simulink model "furuta"  (R2025b)
settings: Solver=VariableStepAuto  StartTime=0.0  StopTime=5  FixedStep=0.01  MaxStep=0.01  RelTol=1e-3
values from neighbouring files (symbols this model uses):
  A_i = double( subs( A_i, subs_array(:,1), subs_array(:,2) ) )    [define_dynamics.m]    (also in dynamics.mat = [0 0 0 0 0 0 0 0 74.6600956651 148.711425653 0 0 ... (25 ele)
  A_s = double( subs( A_s, subs_array(:,1), subs_array(:,2) ) )    [define_dynamics.m]    (also in dynamics.mat = [0 0 0 0 0 0 0 0 74.6600956651 -148.711425653 0 0 ... (25 el)
  Abig_i = [ A_i-B_i*K_i          , B_i*K_i ... (first row only)    [create_inverted_ctrl.m]
  B_i = double( subs( B_i, subs_array(:,1), subs_array(:,2) ) )    [define_dynamics.m]    (also in dynamics.mat = [0 0 625 0 0])
  B_s = double( subs( B_s, subs_array(:,1), subs_array(:,2) ) )    [define_dynamics.m]    (also in dynamics.mat = [0 0 625 0 0])
  C = eye( 5, 5 )    [define_dynamics.m]    (also in dynamics.mat = [1 0 0 0 0 0 1 0 0 0 0 0 ... (25 elements, 5x5)])
  C_i = [ 1 0 0 0 0 ... (first row only)    [create_inverted_ctrl.m]    (also in create_inverted_ctrl_dt.m)
  C_s = [ 0 ]    [analyze_linear_dynamics.m]    (also in create_suspended_ctrl.m = [1 0 0 0 0; create_suspended_ctrl_dt.m = [ 1 0 0 0 0; simulink_companion.m = [ 1 0 0 0 0)
  D = zeros( 5, 1 )    [define_dynamics.m]    (also in dynamics.mat = [0 0 0 0 0])
  D_s = zeros(3,1)    [create_suspended_ctrl.m]    (also in create_suspended_ctrl_dt.m = [ 0; simulink_companion.m = zeros( 3, 5 ))
  K_i = place( A_i, B_i, p )    [create_inverted_ctrl.m]    (also in create_inverted_ctrl_dt.m = place( A_i, B_i, pc ))
  K_s = place( A_s, B_s, p )    [analyze_linear_dynamics.m]    (also in create_suspended_ctrl.m = place( A_s, B_s, pc ); simulink_companion.m)
  K_s_nl = K_s    [simulink_companion.m]
  L_i = place( A_i', C_i', p )'    [create_inverted_ctrl.m]    (also in create_inverted_ctrl_dt.m = place( A_i', C_i', po )')
  L_s = place( A_s', C_s', po )'    [create_suspended_ctrl.m]    (also in simulink_companion.m = place( A_s', C_s', p )')
libraries: simulink x1
settings Model: Creator=shara  LastModifiedBy=shara

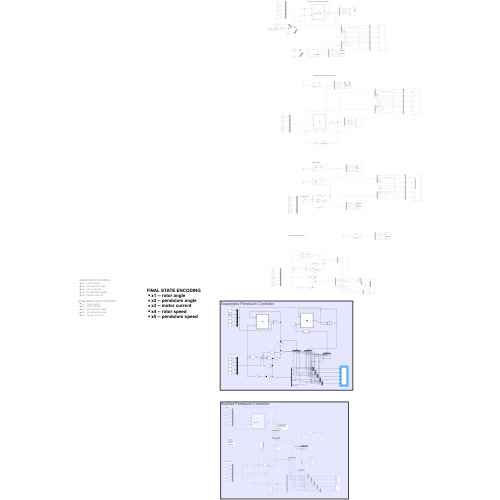
[thumbnail: Simulink's stored preview of the top-level diagram]
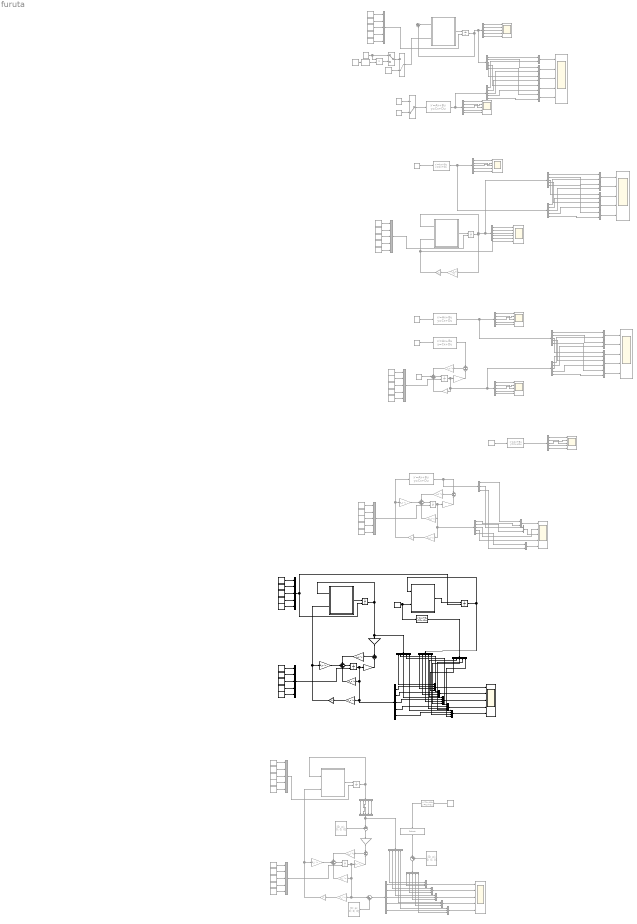
== system furuta ==
  note: $\tilde{x} = x - x_\text{eq}$
  note: LINEAR STATE ENCODING
      | x1 -- rotor angle
      | x2 -- pendulum angle
      | x3 -- rotor speed
      | x4 -- pendulum speed
      | x5 -- motor current
      |
      | NONLINEAR STATE ENCODING
      | x1 -- rotor angle
      | x2 -- rotor speed
      | x3 -- pendulum angle
      | x4 -- pendulum speed
      | x5 -- motor current
  note: NOTE: V_eq = 0, so we don't have to adjust the pertubation
  note: Suspended Pendulum Controller
  note: Observer ICs
  note: State ICs
  note: Combined controller and observer
  note: Zero input for now
  note: Observer design
  note: State feedback controller applied to linear system
  note: make sure to load dynamics.mat to workspace
  note: Inverted Pendulum Controller
  note: flip ordering of states (nonlinear and ss reps have different orderings)
  note: Observer ICs
  note: State ICs
  note: FINAL STATE ENCODING
      | x1 -- rotor angle
      | x2 -- pendulum angle
      | x3 -- motor current
      | x4 -- rotor speed
      | x5 -- pendulum speed
  Constant{,2..4,7..8,10,12..23,25..28,39..43,45..47} (31 alike) : Constant  Commented=on  Value=0
  Constant1 : Constant  Commented=on  Value=0.1
  Constant11 : Constant  Commented=on  Value=1.4
  Constant24 : Constant  Commented=on  Value=0.1
  Constant{9,29..32,34..37} (9 alike) : Constant  Value=0
  Constant33 : Constant  Value=0.1
  Constant44 : Constant  Commented=on  Value=pi + 0.4
  Constant48 : Constant  Commented=on  Value=0.4
  Constant5 : Constant  Commented=on  Value=0.8
  Constant6 : Constant  Commented=on  Value=9
  Demux{,1..12,15,18..21} (18 alike) : Demux  Commented=on  Outputs=5
  Demux13 : Demux  Commented=on  Outputs=3
  Demux{14,16..17,22} (4 alike) : Demux  Outputs=5
  Gain : Gain  Commented=on  Gain=-1
  Gain1 : Gain  Commented=on  Gain=L_s  Multiplication=Matrix(K*u)
  Gain10 : Gain  Commented=on  Gain=-1
  Gain11 : Gain  Gain=-1
  Gain12 : Gain  Gain=L_s  Multiplication=Matrix(K*u)
  Gain13 : Gain  Gain=C_s  Multiplication=Matrix(K*u)
  Gain14 : Gain  Gain=A_s  Multiplication=Matrix(K*u)
  Gain15 : Gain  Gain=K_s  Multiplication=Matrix(K*u)
  Gain16 : Gain  Gain=B_s  Multiplication=Matrix(K*u)
  Gain17 : Gain  Gain=C_s  Multiplication=Matrix(K*u)
  Gain18 : Gain  Commented=on  Gain=-1
  Gain19 : Gain  Commented=on  Gain=L_i  Multiplication=Matrix(K*u)
  Gain2 : Gain  Commented=on  Gain=C_s  Multiplication=Matrix(K*u)
  Gain20 : Gain  Commented=on  Gain=C_i  Multiplication=Matrix(K*u)
  Gain21 : Gain  Commented=on  Gain=A_i  Multiplication=Matrix(K*u)
  Gain22 : Gain  Commented=on  Gain=K_i  Multiplication=Matrix(K*u)
  Gain23 : Gain  Commented=on  Gain=B_i  Multiplication=Matrix(K*u)
  Gain24 : Gain  Commented=on  Gain=C_i  Multiplication=Matrix(K*u)
  Gain3 : Gain  Commented=on  Gain=A_s  Multiplication=Matrix(K*u)
  Gain4 : Gain  Commented=on  Gain=K_s_nl  Multiplication=Matrix(K*u)
  Gain5 : Gain  Commented=on  Gain=L_s  Multiplication=Matrix(K*u)
  Gain6 : Gain  Commented=on  Gain=C_s  Multiplication=Matrix(K*u)
  Gain7 : Gain  Commented=on  Gain=A_s  Multiplication=Matrix(K*u)
  Gain8 : Gain  Commented=on  Gain=K_s  Multiplication=Matrix(K*u)
  Gain9 : Gain  Commented=on  Gain=B_s  Multiplication=Matrix(K*u)
  Integrator{,1..3,6..7} (6 alike) : Integrator  Commented=on  InitialConditionSource=external
  Integrator4 : Integrator  InitialConditionSource=external
  Integrator5 : Integrator  InitialConditionSource=external
  Integrator8 : Integrator  InitialConditionSource=external
  MATLAB Function : MATLAB Function  Commented=on  TreatAsAtomicUnit=on
  MATLAB Function1 : MATLAB Function  Commented=on  TreatAsAtomicUnit=on
  MATLAB Function2 : MATLAB Function  TreatAsAtomicUnit=on
  MATLAB Function3 : MATLAB Function  Commented=on  TreatAsAtomicUnit=on
  MATLAB Function4 : MATLAB Function  TreatAsAtomicUnit=on
  Manual Switch : ManualSwitch  Commented=on
  Manual Switch1 : ManualSwitch  Commented=on  CurrentSetting=0
  Manual Switch2 : ManualSwitch  Commented=on  CurrentSetting=0
  Mux{,6,12,18,30,34..35} (7 alike) : Mux  Commented=on  Inputs=5
  Mux{1..5,7..11,13..17,19..21} (18 alike) : Mux  Commented=on  Inputs=2
  Mux22 : Mux  Inputs=5
  Mux{23..25,28..29} (5 alike) : Mux
  Mux26 : Mux  Inputs=5
  Mux{31..33,36..37} (5 alike) : Mux  Commented=on  Inputs=3
  PWM : simulink/Discontinuities/PWM  Commented=on  DisableCoverage=on  Period=1  InitialDelay=0  DisallowZeroDutyCycle=off  RunAtFixedTimeIntervals=off  SampleTime=0.1
  Product : Product  Commented=on
  Scope{,1..3,5..9,11,13} (11 alike) : Scope  Commented=on  NumInputPorts=5
      Scope settings: ActiveDisplayYMinimum=-3.7270242046645028  ActiveDisplayYMaximum=33.543217841980535
      Scope1 settings: ActiveDisplayYMinimum=-117.90303663058175  ActiveDisplayYMaximum=1061.1273296752361
      Scope11 settings: ActiveDisplayYMinimum=-0.290403063079641  ActiveDisplayYMaximum=0.034920761897079544  DataLoggingVariableName=ScopeData11
      Scope13 settings: ActiveDisplayYMinimum=-259.86893122586537  ActiveDisplayYMaximum=2338.8203810327886  DataLoggingVariableName=ScopeData13
      Scope2 settings: ActiveDisplayYMinimum=-0.0039482366104553225  ActiveDisplayYMaximum=0.018438819297302636  DataLoggingVariableName=ScopeData2
      Scope3 settings: ActiveDisplayYMinimum=-4.0656804845702812  ActiveDisplayYMaximum=0.488883591742888  DataLoggingVariableName=ScopeData3
      Scope5 settings: ActiveDisplayYMinimum=-4.0656463829651983  ActiveDisplayYMaximum=0.48889649908749061  DataLoggingVariableName=ScopeData5
      Scope6 settings: ActiveDisplayYMinimum=-117.90303663058175  ActiveDisplayYMaximum=1061.1273296752361  DataLoggingVariableName=ScopeData6
      Scope7 settings: ActiveDisplayYMinimum=-0.004185188614979185  ActiveDisplayYMaximum=0.035832011704595886  DataLoggingVariableName=ScopeData7
      Scope8 settings: ActiveDisplayYMinimum=-0.0022318445715274631  ActiveDisplayYMaximum=0.018248459199325207  DataLoggingVariableName=ScopeData8
      Scope9 settings: ActiveDisplayYMinimum=-1.3770912495701249  ActiveDisplayYMaximum=0.889510098113746  DataLoggingVariableName=ScopeData9
  Scope10 : Scope  NumInputPorts=5
      settings: ActiveDisplayYMinimum=-0.12968524749349708  ActiveDisplayYMaximum=0.021578200208366552  DataLoggingVariableName=ScopeData10
  Scope4 : Scope  Commented=on  NumInputPorts=6
      settings: ActiveDisplayYMinimum=-2.8540565838343048  ActiveDisplayYMaximum=0.34750097279045905  DataLoggingVariableName=ScopeData4
  Selector : Selector  Commented=on  InputPortWidth=10  IndexOptions=Index vector (dialog)  Indices=[1:5]  OutputSizes=1
  State-Space : StateSpace  Commented=on  A=A_s  B=B_s  C=C  D=D  InitialCondition=[0 0.1 0 0 0];
  State-Space1 : StateSpace  Commented=on  A=A_s -B_s*K_s  B=zeros(5,1)  C=C  D=D  InitialCondition=[0 1.4 0 0 0]
  State-Space2 : StateSpace  Commented=on  A=A_s  B=B_s  C=C_s  D=D_s  InitialCondition=[0 0.1 0 0 0];
  State-Space3 : StateSpace  Commented=on  A=A_s  B=B_s  C=C  D=D  InitialCondition=[0 0.1 0 0 0];
  State-Space4 : StateSpace  Commented=on  A=A_s  B=B_s  C=C_s  D=D_s  InitialCondition=[0 1.4 0 0 0];
  State-Space5 : StateSpace  Commented=on  A=Abig_i  B=zeros(10,1)  C=[ eye(5), zeros(5); zeros(5), zeros(5) ]  D=zeros(10,1)  InitialCondition=[0; 0.01; 0; 0; 0; 0; 0; 0; 0; 0]
  State-Space6 : StateSpace  Commented=on  A=A_s -B_s*K_s  B=zeros(5,1)  C=C  D=D  InitialCondition=[0 0.1 0 0 0]
  State-Space7 : StateSpace  A=A_s  B=B_s  C=eye(5)  D=zeros(5,1)  InitialCondition=[0; 0.1; 0; 0; 0]
  Sum : Sum  Commented=on  Inputs=|++
  Sum1 : Sum  Commented=on  Inputs=+++
  Sum10 : Sum  Commented=on  Inputs=|++
  Sum11 : Sum  Commented=on  Inputs=|++
  Sum2 : Sum  Commented=on  Inputs=+|-
  Sum3 : Sum  Commented=on  Inputs=+++
  Sum4 : Sum  Commented=on  Inputs=+|-
  Sum5 : Sum  Inputs=+++
  Sum6 : Sum  Inputs=+|-
  Sum7 : Sum  Commented=on  Inputs=+++
  Sum8 : Sum  Commented=on  Inputs=+|-
  Sum9 : Sum  Commented=on  Inputs=-+|
  Zero : Constant  Commented=on  Value=0  OutDataTypeStr=Inherit: Inherit via back propagation
  Zero1 : Constant  Commented=on  Value=9  OutDataTypeStr=Inherit: Inherit via back propagation
  Zero2 : Constant  Commented=on  Value=0  OutDataTypeStr=Inherit: Inherit via back propagation
  Zero3 : Constant  Value=0  OutDataTypeStr=Inherit: Inherit via back propagation
  x_eq : Constant  Commented=on  Value=[0; pi; 0; 0; 0]  VectorParams1D=off
  x_eq1 : Constant  Commented=on  Value=[0; pi; 0; 0; 0]  VectorParams1D=off
  x_eq2 : Constant  Commented=on  Value=[0; pi; 0; 0; 0]  VectorParams1D=off
  wires:
  MATLAB Function/1(dx) -> Integrator/1
  Sum/1 -> MATLAB Function/1(x)
  Demux/1 -> Scope/1  "theta_1"
  Demux/2 -> Scope/2  "theta_1_dot"
  Demux/3 -> Scope/3  "theta_2"
  Demux/4 -> Scope/4  "theta_2_dot"
  Constant/1 -> Mux/2
  Constant1/1 -> Mux/3
  Constant2/1 -> Mux/4
  Constant3/1 -> Mux/5
  Constant4/1 -> Mux/1
  Demux/5 -> Scope/5  "i"
  Zero1/1 -> Product/1, Manual Switch/1
  Constant5/1 -> PWM/1
  PWM/1 -> Product/2
  Product/1 -> Manual Switch/2
  State-Space/1 -> Demux2/1, Demux1/1
  Demux1/4 -> Scope1/4  "theta_2_dot"
  Demux1/2 -> Scope1/3  "theta_2"
  Demux1/3 -> Scope1/2  "theta_1_dot"
  Demux1/5 -> Scope1/5  "i"
  Demux1/1 -> Scope1/1  "theta_1"
  Demux2/5 -> Mux5/2  "i"
  Demux2/4 -> Mux4/2  "theta_2_dot"
  Demux2/1 -> Mux1/2  "theta_1 (LINEAR)"
  Demux2/2 -> Mux3/2  "theta_2"
  Demux2/3 -> Mux2/2  "theta_1_dot"
  Demux3/4 -> Mux4/1  "theta_2_dot"
  Demux3/2 -> Mux2/1  "theta_1_dot"
  Demux3/3 -> Mux3/1  "theta_2"
  Demux3/5 -> Mux5/1  "i"
  Demux3/1 -> Mux1/1  "theta_1"
  Integrator/1 -> Demux3/1, Demux/1, Sum/2
  Mux1/1 -> Scope2/1
  Mux2/1 -> Scope2/2
  Mux3/1 -> Scope2/3
  Mux4/1 -> Scope2/4
  Mux5/1 -> Scope2/5
  Demux4/1 -> Scope3/1  "theta_1"
  Demux4/4 -> Scope3/4  "theta_2_dot"
  Demux4/2 -> Scope3/3  "theta_2"
  Demux4/3 -> Scope3/2  "theta_1_dot"
  Demux4/5 -> Scope3/5  "i"
  Constant7/1 -> State-Space1/1
  MATLAB Function1/1(dx) -> Integrator1/1
  Gain4/1 -> Gain/1
  Demux5/2 -> Scope4/2  "theta_1_dot"
  Demux5/3 -> Scope4/3  "theta_2"
  Demux5/5 -> Scope4/5  "i"
  Demux5/4 -> Scope4/4  "theta_2_dot"
  Demux5/1 -> Scope4/1  "theta_1"
  Constant13/1 -> Mux6/5
  Constant11/1 -> Mux6/3
  Constant12/1 -> Mux6/4
  Constant14/1 -> Mux6/1
  Constant10/1 -> Mux6/2
  Gain/1 -> MATLAB Function1/2(V), Scope4/6  "V_in"
  Mux6/1 -> Integrator1/2
  Zero2/1 -> Manual Switch1/2
  Manual Switch/1 -> Manual Switch1/1
  Manual Switch1/1 -> MATLAB Function/2(V)
  Constant6/1 -> Manual Switch2/1
  Constant8/1 -> Manual Switch2/2
  Manual Switch2/1 -> State-Space/1
  Mux/1 -> Integrator/2
  Mux8/1 -> Scope5/2
  Integrator1/1 -> Gain4/1, MATLAB Function1/1(x), Demux7/1, Demux5/1
  Demux7/2 -> Mux8/1  "theta_1_dot"
  Demux7/5 -> Mux11/1  "i"
  Demux7/1 -> Mux7/1  "theta_1"
  Demux6/2 -> Mux9/2  "theta_2"
  Demux6/4 -> Mux10/2  "theta_2_dot"
  Demux6/1 -> Mux7/2  "theta_1 (LINEAR)"
  Mux9/1 -> Scope5/3
  Demux7/4 -> Mux10/1  "theta_2_dot"
  Demux6/3 -> Mux8/2  "theta_1_dot"
  Mux11/1 -> Scope5/5
  Demux7/3 -> Mux9/1  "theta_2"
  Mux10/1 -> Scope5/4
  State-Space1/1 -> Demux6/1, Demux4/1
  Mux7/1 -> Scope5/1
  Demux6/5 -> Mux11/2  "i"
  Constant15/1 -> State-Space3/1
  State-Space3/1 -> Demux11/1, Demux8/1
  Constant16/1 -> State-Space2/1
  Demux8/3 -> Scope6/2  "theta_1_dot"
  Demux8/4 -> Scope6/4  "theta_2_dot"
  Demux8/5 -> Scope6/5  "i"
  Demux8/2 -> Scope6/3  "theta_2"
  Demux8/1 -> Scope6/1  "theta_1"
  Sum2/1 -> Gain1/1
  Gain1/1 -> Sum1/1
  State-Space2/1 -> Sum2/1
  Constant17/1 -> Sum1/2
  Sum1/1 -> Integrator2/1
  Gain2/1 -> Sum2/2
  Gain3/1 -> Sum1/3
  Constant20/1 -> Mux12/4
  Constant19/1 -> Mux12/3
  Constant22/1 -> Mux12/1
  Constant18/1 -> Mux12/2
  Constant21/1 -> Mux12/5
  Mux12/1 -> Integrator2/2
  Demux9/2 -> Scope7/3  "theta_2"
  Demux9/5 -> Scope7/5  "i"
  Integrator2/1 -> Gain2/1, Demux10/1, Demux9/1, Gain3/1
  Demux9/4 -> Scope7/4  "theta_2_dot"
  Demux9/3 -> Scope7/2  "theta_1_dot"
  Demux9/1 -> Scope7/1  "theta_1"
  Mux15/1 -> Scope8/1
  Demux10/5 -> Mux14/2  "i"
  Mux13/1 -> Scope8/4
  Demux10/4 -> Mux13/2  "theta_2_dot"
  Mux14/1 -> Scope8/5
  Demux11/3 -> Mux17/1  "theta_1_dot"
  Demux10/3 -> Mux17/2  "theta_1_dot"
  Demux10/2 -> Mux16/2  "theta_2"
  Mux17/1 -> Scope8/3
  Demux11/2 -> Mux16/1  "theta_2"
  Demux11/4 -> Mux13/1  "theta_2_dot"
  Mux16/1 -> Scope8/2
  Demux10/1 -> Mux15/2  "theta_1 (FROM OBSERVER)"
  Demux11/1 -> Mux15/1  "theta_1"
  Demux11/5 -> Mux14/1  "i"
  Gain5/1 -> Sum3/1
  Gain9/1 -> Sum3/2
  Gain7/1 -> Sum3/3
  Gain8/1 -> Gain10/1
  Sum3/1 -> Integrator3/1
  Gain6/1 -> Sum4/2
  Integrator3/1 -> Demux12/1, Gain8/1, Gain7/1, Gain6/1
  Constant25/1 -> Mux18/3
  Constant27/1 -> Mux18/5
  Constant28/1 -> Mux18/1
  Constant24/1 -> Mux18/2
  Constant26/1 -> Mux18/4
  Sum4/1 -> Gain5/1
  State-Space4/1 -> Demux13/1, Sum4/1
  Mux18/1 -> Integrator3/2
  Demux12/3 -> Scope9/2  "theta_1_dot"
  Demux12/4 -> Scope9/4  "theta_2_dot"
  Demux12/1 -> Mux19/2  "theta_1"
  Demux12/5 -> Mux21/1  "i"
  Demux12/2 -> Mux20/2  "theta_2"
  Gain10/1 -> State-Space4/1, Gain9/1
  Demux13/1 -> Mux19/1  "theta_1"
  Demux13/2 -> Mux20/1  "theta_2"
  Demux13/3 -> Mux21/2  "i"
  Mux20/1 -> Scope9/3
  Mux19/1 -> Scope9/1
  Mux21/1 -> Scope9/5
  Demux15/1 -> Scope11/1  "theta_1"
  Demux15/2 -> Scope11/3  "theta_2"
  State-Space6/1 -> Demux15/1
  Demux15/4 -> Scope11/4  "theta_2_dot"
  Constant23/1 -> State-Space6/1
  Demux15/3 -> Scope11/2  "theta_1_dot"
  Demux15/5 -> Scope11/5  "i"
  Demux14/3 -> Mux29/2  "i"
  Mux22/1 -> Integrator4/2
  Constant29/1 -> Mux22/3
  Constant30/1 -> Mux22/4
  Sum6/1 -> Gain12/1
  Constant9/1 -> Mux22/2
  Mux24/1 -> Scope10/2
  Constant31/1 -> Mux22/5
  Constant32/1 -> Mux22/1
  Gain13/1 -> Sum6/2
  Sum5/1 -> Integrator4/1
  Gain12/1 -> Sum5/1
  Demux14/2 -> Mux24/2  "theta_2"
  Mux25/1 -> Scope10/5
  Integrator4/1 -> Gain13/1, Demux14/1, Gain15/1, Gain14/1
  Gain16/1 -> Sum5/2
  Gain14/1 -> Sum5/3
  Gain15/1 -> Gain11/1
  Demux14/1 -> Mux23/2  "theta_1"
  Demux14/4 -> Mux28/2  "theta_1_dot"
  Mux23/1 -> Scope10/1
  Demux14/5 -> Mux25/2  "theta_2_dot"
  Gain11/1 -> MATLAB Function2/2(V), Gain16/1
  MATLAB Function2/1(dx) -> Integrator5/1
  Constant33/1 -> Mux26/2
  Constant37/1 -> Mux26/1
  Constant36/1 -> Mux26/5
  Constant34/1 -> Mux26/3
  Constant35/1 -> Mux26/4
  Mux26/1 -> Integrator8/2, Integrator5/2
  Gain17/1 -> Sum6/1
  Integrator5/1 -> Demux16/1, Gain17/1, MATLAB Function2/1(x)
  Demux16/1 -> Mux23/1  "theta_1 (GROUND TRUTH)"
  Demux16/2 -> Mux24/1  "theta_2"
  Demux16/3 -> Mux29/1  "i"
  Demux16/4 -> Mux28/1  "theta_1_d"
  Demux16/5 -> Mux25/1  "theta_2_dot"
  Mux28/1 -> Scope10/4
  Mux29/1 -> Scope10/3
  State-Space5/1 -> Selector/1
  Sum7/1 -> Integrator6/1
  Mux35/1 -> Sum9/2, Demux20/1
  Gain22/1 -> Gain18/1
  Constant44/1 -> Mux34/3
  Mux33/1 -> Scope13/5
  Demux19/5 -> Mux33/2  "i"
  Gain24/1 -> Sum8/1
  Mux32/1 -> Scope13/2
  Gain21/1 -> Sum7/3
  Demux19/2 -> Mux32/2  "theta_2"
  Demux20/1 -> Mux31/1  "theta_1 (GROUND TRUTH)"
  Demux19/1 -> Mux31/2  "theta_1"
  Integrator6/1 -> Gain20/1, Sum10/1, Gain22/1, Gain21/1
  Demux21/1 -> Mux35/1  "t1"
  Demux20/3 -> Mux37/1  "theta_1_d"
  Constant40/1 -> Mux30/4
  Demux20/5 -> Mux33/1  "i"
  MATLAB Function3/1(dx) -> Integrator7/1
  Demux19/4 -> Mux36/2  "theta_2_dot"
  Demux21/5 -> Mux35/5  "i"
  Demux20/4 -> Mux36/1  "theta_2_d"
  Constant48/1 -> Mux30/2
  Mux37/1 -> Scope13/3
  Mux36/1 -> Scope13/4
  Constant47/1 -> Mux34/1
  Constant46/1 -> Mux34/5
  Sum8/1 -> Gain19/1
  Gain20/1 -> Sum8/2
  Demux21/3 -> Mux35/2  "t2"
  Gain19/1 -> Sum7/1
  Constant39/1 -> Mux30/3
  Constant42/1 -> Mux30/1
  Gain23/1 -> Sum7/2
  Demux21/2 -> Mux35/3  "t1d"
  Gain18/1 -> MATLAB Function3/2(V), Gain23/1
  Demux21/4 -> Mux35/4  "t2d"
  Demux20/2 -> Mux32/1  "theta_2"
  Mux30/1 -> Integrator6/2
  Demux19/3 -> Mux37/2  "theta_1_dot"
  Mux34/1 -> Integrator7/2
  Mux31/1 -> Scope13/1
  Constant45/1 -> Mux34/4
  Constant41/1 -> Mux30/5
  Integrator7/1 -> Demux21/1, MATLAB Function3/1(x)
  Constant43/1 -> Mux34/2
  Sum9/1 -> Gain24/1
  x_eq/1 -> Sum9/1
  Sum10/1 -> Demux19/1
  x_eq1/1 -> Sum10/2
  Zero/1 -> State-Space5/1
  x_eq2/1 -> Sum11/2
  Sum11/1 -> Demux18/1
  Demux18/1 -> Mux31/3
  Demux18/2 -> Mux32/3
  Demux18/3 -> Mux37/3
  Demux18/4 -> Mux36/3
  Demux18/5 -> Mux33/3
  Selector/1 -> Sum11/1
  Zero3/1 -> State-Space7/1, MATLAB Function4/2(V)
  MATLAB Function4/1(dx) -> Integrator8/1
  Integrator8/1 -> Demux17/1, MATLAB Function4/1(x)
  Demux17/1 -> Mux23/3  "theta_1 (GROUND TRUTH)"
  Demux17/2 -> Mux24/3  "theta_2"
  Demux17/3 -> Mux29/3  "i"
  Demux17/4 -> Mux28/3  "theta_1_d"
  Demux17/5 -> Mux25/3  "theta_2_dot"
  State-Space7/1 -> Demux22/1
  Demux22/1 -> Mux23/4  "theta_1 (GROUND TRUTH)"
  Demux22/2 -> Mux24/4  "theta_2"
  Demux22/3 -> Mux29/4  "i"
  Demux22/4 -> Mux28/4  "theta_1_d"
  Demux22/5 -> Mux25/4  "theta_2_dot"

== matlab function furuta/MATLAB Function1 ==
  data: x input; dx output; V input
function dx = nonlinear_furuta(x, V)

dx = simulate_dynamics_func( x, V );

== matlab function furuta/MATLAB Function ==
  data: x input; dx output; V input
function dx = nonlinear_furuta(x, V)

dx = simulate_dynamics_func( x, V );

== matlab function furuta/MATLAB Function2 ==
  data: x input; dx output; V input
function dx = nonlinear_furuta(x, V)

dx = simulate_dynamics_func( x, V );

== matlab function furuta/MATLAB Function3 ==
  data: x input; dx output; V input
function dx = nonlinear_furuta(x, V)

dx = simulate_dynamics_func( x, V );

== matlab function furuta/MATLAB Function4 ==
  data: x input; dx output; V input
function dx = nonlinear_furuta(x, V)

dx = simulate_dynamics_func( x, V );
